simulink model "Gesamt"  (R2015b)
settings: Solver=ode3  SolverMode=SingleTasking  StartTime=0.0  StopTime=inf  RelTol=1e-3
InitFcn:
  | Reglerauslegung
values from neighbouring files (symbols this model uses):
  aMax = 498    [Reglerauslegung.m]
  aMaxPsi = 1    [Reglerauslegung.m]
  Blindzeit = 25    [Reglerauslegung.m]
  dt = 0.005    [Reglerauslegung.m]
  K1 = place(AI1,BI1,pWunschI1)    [Reglerauslegung.m]
  K2 = place(A2,B2,pWunsch2)    [Reglerauslegung.m]
  K3 = place(A3,B3,pWunsch3)    [Reglerauslegung.m]
  Kx = 0.9575    [Reglerauslegung.m]
  Ky = 0.9575    [Reglerauslegung.m]
  Tx = 1/4.1668    (= 0.239992320246)    [Reglerauslegung.m]
  Ty = 1/4.1668    (= 0.239992320246)    [Reglerauslegung.m]
  vMax = 403    [Reglerauslegung.m]
  vMaxPsi = 3    [Reglerauslegung.m]
undefined symbols (not defined in the file or in its folder): sigbuilder_block
libraries: simulink x5, xpcutilitieslib x1
(part 1 of 3)
CloseFcn:
  | rtwprivate ssgencode ModelCloseRequest Robotino_Strecke_reall_2009
settings Model: SimulationMode=external  Creator=atlabor  LastModifiedBy=atlabor
settings SolverCC: EnableConcurrentExecution=on
settings DataIOCC: SignalLoggingSaveFormat=ModelDataLogs
settings OptimizationCC: BlockReduction=off  OptimizeBlockIOStorage=off  BufferReuse=off  GlobalBufferReuse=off  ExpressionFolding=off  ExpressionDepthLimit=2147483647  LocalBlockOutputs=off  InitFltsAndDblsToZero=on
settings DebuggingCC: SaveWithParameterizedLinksMsg=none  UnderspecifiedInitializationDetection=Classic  MergeDetectMultiDrivingBlocksExec=none  SolverPrmCheckMsg=warning  FcnCallInpInsideContextMsg=EnableAllAsWarning  StateNameClashWarn=warning
settings HardwareCC: ProdBitPerPointer=32  ProdLargestAtomicFloat=None  ProdWordSize=32  ProdLongLongMode=on  ProdHWDeviceType=Generic->32-bit x86 compatible
settings SFSimCC: SimParseCustomCode=off
settings RTWCC: SystemTargetFile=TwinCAT.tlc  GenCodeOnly=on  MakeCommand=make_tct  TemplateMakefile=tct_msbuild.tmf  Description=TwinCAT Target  GenerateReport=on  TargetLang=C++
settings STFCustomTargetCC: CompOptLevelCompliant=on  ConcurrentExecutionCompliant=off  GeneratePreprocessorConditionals=Use local settings  MATLABClassNameForMDSCustomization=Simulink.SoftwareTarget.TargetSpecificTriggerConfigurationBase  CPPClassGenCompliant=off  SystemTargetFile=TwinCAT.tlc
settings ConfigComp: CovModelRefEnable=Off  CovSFcnEnable=off

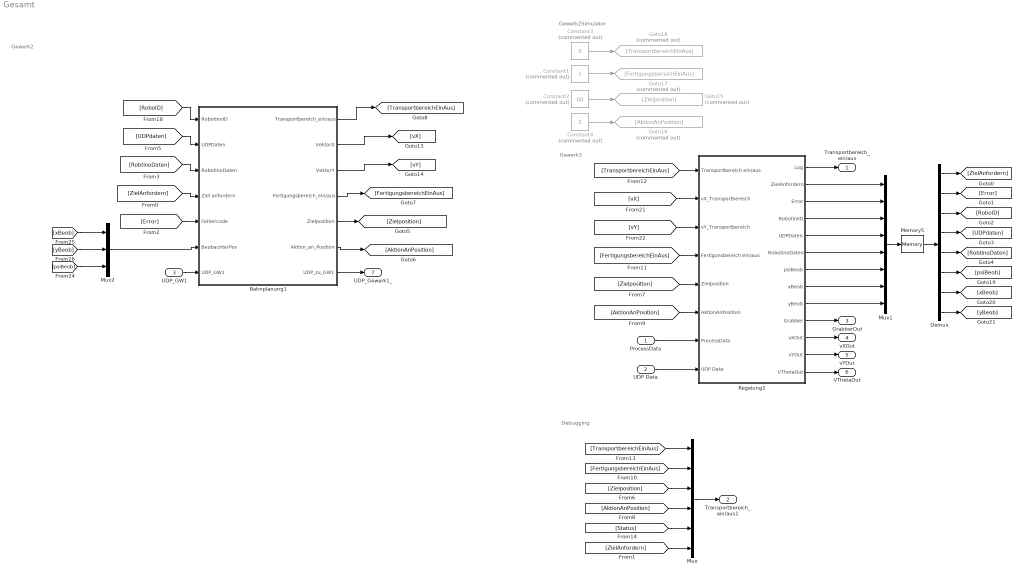
== system Gesamt ==
  note: Gewerk2Simulator
  note: Gewerk3
  note: Gewerk2
  note: Debugging
  ProcessData : Inport
  UDP Data : Inport  Port=2  PortDimensions=56
  UDP_GW1 : Inport  Port=3  PortDimensions=8
  Bahnplanung1 : Subsystem
  Constant1 : Constant  Commented=on
  Constant2 : Constant  Commented=on  Value=60
  Constant3 : Constant  Commented=on  Value=0
  Constant4 : Constant  Commented=on  Value=2
  Demux : Demux  Outputs=8
  Goto15 : Goto  Commented=on  GotoTag=Zielposition
  Goto16 : Goto  Commented=on  GotoTag=AktionAnPosition
  Goto17 : Goto  Commented=on  GotoTag=FertigungsbereichEinAus
  Goto18 : Goto  Commented=on  GotoTag=TransportbereichEinAus
  Memory5 : Memory
  Mux : Mux  Inputs=6
  Mux1 : Mux  Inputs=8
  Mux2 : Mux  Inputs=3
  Regelung1 : Subsystem
  Transportbereich_ein/aus : Outport
  Transportbereich_ein/aus1 : Outport  Port=2
  GrabberOut : Outport  Port=3
  vXOut : Outport  Port=4
  vYOut : Outport  Port=5
  VThetaOut : Outport  Port=6
  UDP_Gewerk1_ : Outport  Port=7
  wires:
  Regelung1/3(Error) -> Mux1/2
  Regelung1/6(RobotinoDaten) -> Mux1/5
  Regelung1/2(ZielAnfordern) -> Mux1/1
  Regelung1/4(RobotiniID) -> Mux1/3
  [ZielAnfordern] -> Mux/6
  Mux1/1 -> Memory5/1
  Demux/1 -> [ZielAnfordern]
  Demux/2 -> [Error]
  Memory5/1 -> Demux/1
  Demux/3 -> [RoboID]
  Demux/4 -> [UDPdaten]
  Regelung1/5(UDPDaten) -> Mux1/4
  Demux/5 -> [RobtinoDaten]
  [Zielposition] -> Mux/3
  [Zielposition] -> Regelung1/5(Zielposition)
  [AktionAnPosition] -> Mux/4
  [AktionAnPosition] -> Regelung1/6(AktionAnPosition)
  [FertigungsbereichEinAus] -> Mux/2
  [FertigungsbereichEinAus] -> Regelung1/4(Fertigunsbereich ein/aus)
  [TransportbereichEinAus] -> Regelung1/1(Transportbereich ein/aus)
  [TransportbereichEinAus] -> Mux/1
  [Status] -> Mux/5
  [RoboID] -> Bahnplanung1/1(RobotinoID)
  [vX] -> Regelung1/2(vX_Transportbereich)
  [vY] -> Regelung1/3(vY_Transportbereich)
  Constant3/1 -> Goto18/1
  Constant1/1 -> Goto17/1
  Constant2/1 -> Goto15/1
  Constant4/1 -> Goto16/1
  Regelung1/7(psiBeob) -> Mux1/6
  Regelung1/8(xBeob) -> Mux1/7
  Regelung1/9(yBeob) -> Mux1/8
  Demux/6 -> [psiBeob]
  Demux/7 -> [xBeob]
  Demux/8 -> [yBeob]
  [psiBeob] -> Mux2/3
  [xBeob] -> Mux2/1
  [yBeob] -> Mux2/2
  Regelung1/1(Log) -> Transportbereich_ein/aus/1
  Mux/1 -> Transportbereich_ein/aus1/1
  [UDPdaten] -> Bahnplanung1/2(UDPDaten)
  [RobtinoDaten] -> Bahnplanung1/3(RobotinoDaten)
  [ZielAnfordern] -> Bahnplanung1/4(Ziel anfordern)
  [Error] -> Bahnplanung1/5(Fehlercode)
  Mux2/1 -> Bahnplanung1/6(BeobachterPos)
  Bahnplanung1/1(Transportbereich_ein/aus) -> [TransportbereichEinAus]
  Bahnplanung1/2(VektorX) -> [vX]
  Bahnplanung1/3("VektorY ") -> [vY]
  Bahnplanung1/4(Fertigungsbereich_ein/aus) -> [FertigungsbereichEinAus]
  Bahnplanung1/5(Zielposition) -> [Zielposition]
  Bahnplanung1/6(Aktion_an_Position) -> [AktionAnPosition]
  ProcessData/1 -> Regelung1/7(ProcessData)
  UDP Data/1 -> Regelung1/8(UDP Data)
  Regelung1/10(Grabber) -> GrabberOut/1
  Regelung1/11(vXOut) -> vXOut/1
  Regelung1/12(vYOut) -> vYOut/1
  Regelung1/13(VThetaOut) -> VThetaOut/1
  Bahnplanung1/7(UDP_zu_GW1) -> UDP_Gewerk1_/1
  UDP_GW1/1 -> Bahnplanung1/7(UDP_GW1)

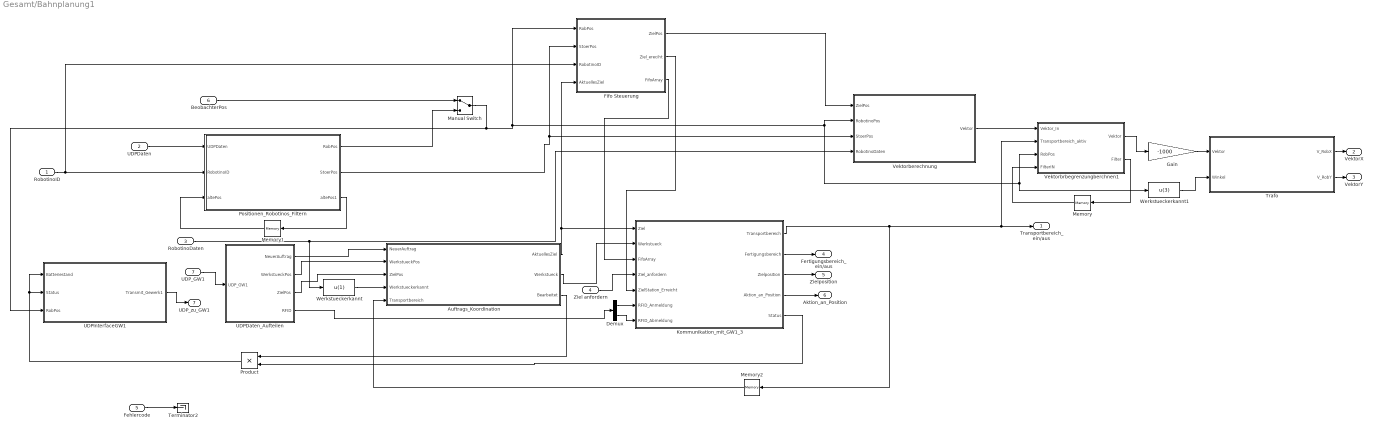
== system Gesamt/Bahnplanung1 ==
  RobotinoID : Inport
  UDPDaten : Inport  Port=2  PortDimensions=56
  RobotinoDaten : Inport  Port=3
  Ziel anfordern : Inport  Port=4
  Fehlercode : Inport  Port=5
  BeobachterPos : Inport  Port=6
  UDP_GW1 : Inport  Port=7  PortDimensions=8
  Auftrags_Koordination : Stateflow chart  TreatAsAtomicUnit=on
  Demux : Demux  Outputs=2
  Fifo Steuerung : Subsystem
  Gain : Gain  Gain=-1000
  Kommunikation_mit_GW1_3 : Stateflow chart  TreatAsAtomicUnit=on
  Manual Switch : ManualSwitch
  Memory : Memory
  Memory1 : Memory
  Memory2 : Memory
  Positionen_Robotinos_Filtern : MATLAB Function  TreatAsAtomicUnit=on
  Product : Product
  Terminator2 : Terminator
  Trafo : MATLAB Function  Tag=Transformation_Global_auf_lokal  TreatAsAtomicUnit=on
  UDPDaten_Aufteilen : Subsystem
  UDPInterfaceGW1 : Subsystem
  Vektorberechnung : Subsystem
  Vektorbrbegrenzungberchnen1 : MATLAB Function  TreatAsAtomicUnit=on
  Werkstueckerkannt : Fcn  Expr=u(1)
  Werkstueckerkannt1 : Fcn  Expr=u(3)
  Transportbereich_ein/aus : Outport
  VektorX : Outport  Port=2  OutDataTypeStr=double
  "VektorY " : Outport  Port=3  OutDataTypeStr=double
  Fertigungsbereich_ein/aus : Outport  Port=4
  Zielposition : Outport  Port=5
  Aktion_an_Position : Outport  Port=6
  UDP_zu_GW1 : Outport  Port=7
  wires:
  RobotinoID/1 -> Positionen_Robotinos_Filtern/2(RobotinoID), Fifo Steuerung/3(RobotinoID)
  UDPDaten/1 -> Positionen_Robotinos_Filtern/1(UDPDaten)
  Positionen_Robotinos_Filtern/2(StoerPos) -> Fifo Steuerung/2(StoerPos), Vektorberechnung/3(StoerPos)
  RobotinoDaten/1 -> Vektorberechnung/4(RobotinoDaten), Werkstueckerkannt/1
  Kommunikation_mit_GW1_3/3(Zielposition) -> Zielposition/1
  Kommunikation_mit_GW1_3/4(Aktion_an_Position) -> Aktion_an_Position/1
  Kommunikation_mit_GW1_3/2(Fertigungsbereich) -> Fertigungsbereich_ein/aus/1
  Kommunikation_mit_GW1_3/1(Transportbereich) -> Memory2/1, Vektorbrbegrenzungberchnen1/2(Transportbereich_aktiv), Transportbereich_ein/aus/1
  UDP_GW1/1 -> UDPDaten_Aufteilen/1(UDP_GW1)
  UDPDaten_Aufteilen/2(WerkstueckPos) -> Auftrags_Koordination/2(WerkstueckPos)
  UDPDaten_Aufteilen/3(ZielPos) -> Auftrags_Koordination/3(ZielPos)
  Auftrags_Koordination/1(AktuellesZiel) -> Fifo Steuerung/4(AktuellesZiel), Kommunikation_mit_GW1_3/1(Ziel)
  Fehlercode/1 -> Terminator2/1
  UDPDaten_Aufteilen/1(NeuerAuftrag) -> Auftrags_Koordination/1(NeuerAuftrag)
  Auftrags_Koordination/2(Werkstueck) -> Kommunikation_mit_GW1_3/2(Werkstueck)
  Werkstueckerkannt/1 -> Auftrags_Koordination/4(Werkstueckerkannt)
  Vektorbrbegrenzungberchnen1/1(Vektor) -> Gain/1
  Gain/1 -> Trafo/1(Vektor)
  Manual Switch/1 -> UDPInterfaceGW1/3(RobPos), Fifo Steuerung/1(RobPos), Vektorbrbegrenzungberchnen1/3(RobPos), Werkstueckerkannt1/1, Vektorberechnung/2(RobotinoPos)
  Vektorberechnung/1(Vektor) -> Vektorbrbegrenzungberchnen1/1(Vektor_In)
  Fifo Steuerung/1(ZielPos) -> Vektorberechnung/1(ZielPos)
  Memory2/1 -> Auftrags_Koordination/5(Transportbereich)
  Kommunikation_mit_GW1_3/5(Status) -> Product/2
  Positionen_Robotinos_Filtern/1(RobPos) -> Manual Switch/2
  Trafo/1(V_RobX) -> VektorX/1
  Trafo/2(V_RobY) -> "VektorY "/1
  BeobachterPos/1 -> Manual Switch/1
  Werkstueckerkannt1/1 -> Trafo/2(Winkel)
  Auftrags_Koordination/3(Bearbeitet) -> Product/1
  Product/1 -> UDPInterfaceGW1/1(Batteriestand), UDPInterfaceGW1/2(Status)
  UDPDaten_Aufteilen/4(RFID) -> Demux/1
  Fifo Steuerung/3("FifoArray ") -> Kommunikation_mit_GW1_3/3(FifoArray)
  Ziel anfordern/1 -> Kommunikation_mit_GW1_3/4(Ziel_anfordern)
  Fifo Steuerung/2(Ziel_ereciht) -> Kommunikation_mit_GW1_3/5(ZielStation_Erreicht)
  Demux/1 -> Kommunikation_mit_GW1_3/6(RFID_Anmeldung)
  Demux/2 -> Kommunikation_mit_GW1_3/7(RFID_Abmeldung)
  Vektorbrbegrenzungberchnen1/2(Filter) -> Memory/1
  Memory/1 -> Vektorbrbegrenzungberchnen1/4(FilterIN)
  Positionen_Robotinos_Filtern/3(altePos1) -> Memory1/1
  Memory1/1 -> Positionen_Robotinos_Filtern/3(altePos)
  UDPInterfaceGW1/1(Transmit_Gewerk1) -> UDP_zu_GW1/1

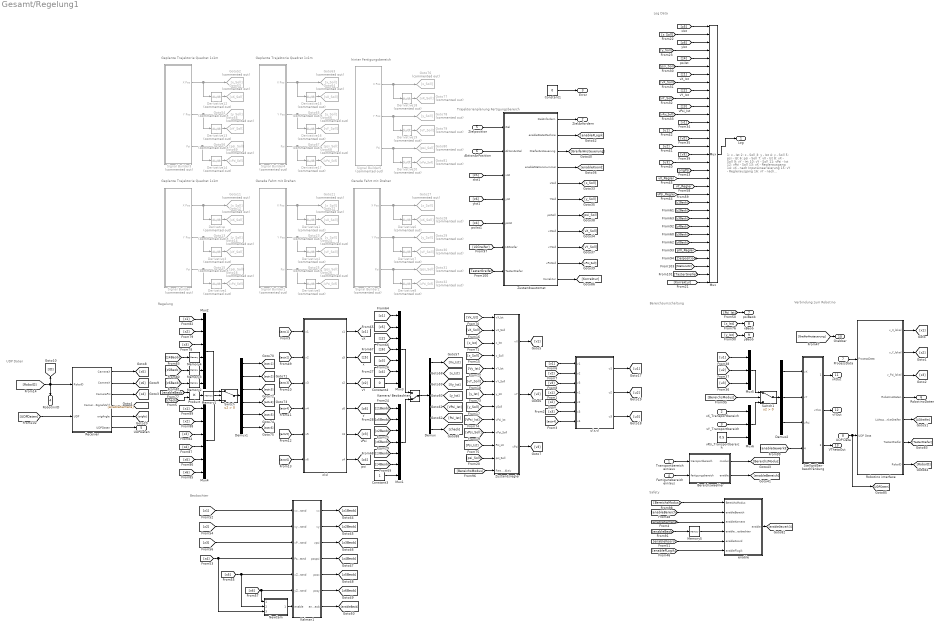
== system Gesamt/Regelung1 ==
  note: Safety
  note: Trajektorienplanung Fertigungsbereich
  note: Regelung
  note: Beobachter
  note: hinter Fertigungsbereich
  note: Geplante Trajektorie Quadrat 1x1m
  note: Geplante Trajektorie Quadrat 1x1m
  note: Gerade Fahrt mit Drehen
  note: Gerade Fahrt mit Drehen
  note: 1:    x     - Ist
      | 2:    x     - Soll
      | 3:    y     - Ist
      | 4:    y     - Soll
      | 5:   psi   - Ist
      | 6:   psi   - Soll
      | 7:   vX   - Ist
      | 8:   vX   - Soll
      | 9:   vY   - Ist
      | 10: vY   - Soll
      | 11: vPsi - Ist
      | 12: vPsi - Soll
      | 13: vX   - Reglerausgang
      | 14: vX   - nach InputLinearisierung
      | 15: vY   - Reglerausgang
      | 16: vY  - nach InputLinearisierung
      | 17: vPsi - Reglerausgang
      | 18: vPsi - nach InputLinearisierung
      | 19: Kamera Psi
      | 20: vX   - Regler (Geschwindigkeit)
      | 21: vY   - Regler (Geschwindigkeit)
      | 22: vPsi - Regler (Geschwindigkeit)
  note: Log Data
  note: Geplante Trajektorie Quadrat 1x1m
  note: UDP Daten
  note: Verbindung zum Robotino
  note: Bereichsumschaltung
  Transportbereich ein/aus : Inport
  vX_Transportbereich : Inport  Port=2
  vY_Transportbereich : Inport  Port=3
  Fertigunsbereich ein/aus : Inport  Port=4
  Zielposition : Inport  Port=5
  AktionAnPosition : Inport  Port=6
  ProcessData : Inport  Port=7
  UDP Data : Inport  Port=8  PortDimensions=56
  Bereichswaehler : MATLAB Function  TreatAsAtomicUnit=on
  Constant1 : Constant  Value=0
  Constant3 : Constant
  Constant4 : Constant  Value=0
  Demux : Demux  Outputs=7
  Demux1 : Demux  Outputs=6
  Demux2 : Demux  Outputs=3
  Derivative{,1..8,12..20} (18 alike) : Derivative  Commented=on
  Goto{11,21,27,52,63,76} (6 alike) : Goto  Commented=on  GotoTag=x_Soll
  Goto{12,22,28,53,64,77} (6 alike) : Goto  Commented=on  GotoTag=vX_Soll
  Goto{13,23,29,54,65,78} (6 alike) : Goto  Commented=on  GotoTag=y_Soll
  Goto{14,24,30,55,66,79} (6 alike) : Goto  Commented=on  GotoTag=vY_Soll
  Goto{15,25,31,56,67,80} (6 alike) : Goto  Commented=on  GotoTag=psi_Soll
  Goto{16,26,32,68..69,81} (6 alike) : Goto  Commented=on  GotoTag=vPsi_Soll
  Kalman1 : MATLAB Function  TreatAsAtomicUnit=on
  Kamera/ Beobachter : ManualSwitch  CurrentSetting=0
  Memory{1..5} (5 alike) : Memory
  Mux : Mux  Inputs=33
  Mux1 : Mux  Inputs=7
  Mux2 : Mux  Inputs=6
  Mux3 : Mux  Inputs=7
  Mux4 : Mux  Inputs=6
  Mux5 : Mux  Inputs=3
  Mux6 : Mux  Inputs=3
  NewCam : MATLAB Function  TreatAsAtomicUnit=on
  Product : Product
  Receiver : Subsystem
  Robotino interface : Subsystem
  Signal Builder : Subsystem  Tag=STV Subsys  Commented=on  LoadFcn=sigbuilder_block('load');  StartFcn=sigbuilder_block('start');  StopFcn=sigbuilder_block('stop');  ClipboardFcn=sigbuilder_block('clipboard');  mask(Sigbuilder block){}
      mask help: Simulink:masks:SigbuilderBlock_MD
      mask init:
      | if ~strcmp(get_param(bdroot(gcbh),'SimulationStatus'),'stopped') tuvar = sigbuilder_block('maskInit'); end
      settings: CopyFcn=sigbuilder_block('copy');  DeleteFcn=sigbuilder_block('delete');  ModelCloseFcn=sigbuilder_block('modelClose');  PreSaveFcn=sigbuilder_block('preSave');  PauseFcn=sigbuilder_block('pause');  ContinueFcn=sigbuilder_block('continue');  NameChangeFcn=sigbuilder_block('namechange');  OpenFcn=sigbuilder_block('open',[6 30 1248 660 ]);  CloseFcn=sigbuilder_block('close');
      mask Display: plot(0, 0, 100, 100,[2, 2, 32, 32, 2], [68, 8, 8, 68, 68],[32, 2], [38, 38], [32, 19, 2],[53, 60, 44], [32, 17, 17, 2],[16, 16, 31, 31]);txt = getActiveGroup(gcbh);text(2, 100, txt,'verticalAlignment', 'top');
  Signal Builder1 : Subsystem  Tag=STV Subsys  Commented=on  LoadFcn=sigbuilder_block('load');  StartFcn=sigbuilder_block('start');  StopFcn=sigbuilder_block('stop');  ClipboardFcn=sigbuilder_block('clipboard');  mask(Sigbuilder block){}
      mask help: Simulink:masks:SigbuilderBlock_MD
      mask init:
      | if ~strcmp(get_param(bdroot(gcbh),'SimulationStatus'),'stopped') tuvar = sigbuilder_block('maskInit'); end
      settings: CopyFcn=sigbuilder_block('copy');  DeleteFcn=sigbuilder_block('delete');  ModelCloseFcn=sigbuilder_block('modelClose');  PreSaveFcn=sigbuilder_block('preSave');  PauseFcn=sigbuilder_block('pause');  ContinueFcn=sigbuilder_block('continue');  NameChangeFcn=sigbuilder_block('namechange');  OpenFcn=sigbuilder_block('open',[6.06316 30.3158 1248.25 659.368 ]);  CloseFcn=sigbuilder_block('close');
      mask Display: plot(0, 0, 100, 100,[2, 2, 32, 32, 2], [68, 8, 8, 68, 68],[32, 2], [38, 38], [32, 19, 2],[53, 60, 44], [32, 17, 17, 2],[16, 16, 31, 31]);txt = getActiveGroup(gcbh);text(2, 100, txt,'verticalAlignment', 'top');
  Signal Builder2 : Subsystem  Tag=STV Subsys  Commented=on  LoadFcn=sigbuilder_block('load');  StartFcn=sigbuilder_block('start');  StopFcn=sigbuilder_block('stop');  ClipboardFcn=sigbuilder_block('clipboard');  mask(Sigbuilder block){}
      mask help: Simulink:masks:SigbuilderBlock_MD
      mask init:
      | if ~strcmp(get_param(bdroot(gcbh),'SimulationStatus'),'stopped') tuvar = sigbuilder_block('maskInit'); end
      settings: CopyFcn=sigbuilder_block('copy');  DeleteFcn=sigbuilder_block('delete');  ModelCloseFcn=sigbuilder_block('modelClose');  PreSaveFcn=sigbuilder_block('preSave');  PauseFcn=sigbuilder_block('pause');  ContinueFcn=sigbuilder_block('continue');  NameChangeFcn=sigbuilder_block('namechange');  OpenFcn=sigbuilder_block('open',[6 30 1248 660 ]);  CloseFcn=sigbuilder_block('close');
      mask Display: plot(0, 0, 100, 100,[2, 2, 32, 32, 2], [68, 8, 8, 68, 68],[32, 2], [38, 38], [32, 19, 2],[53, 60, 44], [32, 17, 17, 2],[16, 16, 31, 31]);txt = getActiveGroup(gcbh);text(2, 100, txt,'verticalAlignment', 'top');
  Signal Builder3 : Subsystem  Tag=STV Subsys  Commented=on  LoadFcn=sigbuilder_block('load');  StartFcn=sigbuilder_block('start');  StopFcn=sigbuilder_block('stop');  ClipboardFcn=sigbuilder_block('clipboard');  mask(Sigbuilder block){}
      mask help: Simulink:masks:SigbuilderBlock_MD
      mask init:
      | if ~strcmp(get_param(bdroot(gcbh),'SimulationStatus'),'stopped') tuvar = sigbuilder_block('maskInit'); end
      settings: CopyFcn=sigbuilder_block('copy');  DeleteFcn=sigbuilder_block('delete');  ModelCloseFcn=sigbuilder_block('modelClose');  PreSaveFcn=sigbuilder_block('preSave');  PauseFcn=sigbuilder_block('pause');  ContinueFcn=sigbuilder_block('continue');  NameChangeFcn=sigbuilder_block('namechange');  OpenFcn=sigbuilder_block('open',[6 30 1248 660 ]);  CloseFcn=sigbuilder_block('close');
      mask Display: plot(0, 0, 100, 100,[2, 2, 32, 32, 2], [68, 8, 8, 68, 68],[32, 2], [38, 38], [32, 19, 2],[53, 60, 44], [32, 17, 17, 2],[16, 16, 31, 31]);txt = getActiveGroup(gcbh);text(2, 100, txt,'verticalAlignment', 'top');
  Signal Builder4 : Subsystem  Tag=STV Subsys  Commented=on  LoadFcn=sigbuilder_block('load');  StartFcn=sigbuilder_block('start');  StopFcn=sigbuilder_block('stop');  ClipboardFcn=sigbuilder_block('clipboard');  mask(Sigbuilder block){}
      mask help: Simulink:masks:SigbuilderBlock_MD
      mask init:
      | if ~strcmp(get_param(bdroot(gcbh),'SimulationStatus'),'stopped') tuvar = sigbuilder_block('maskInit'); end
      settings: CopyFcn=sigbuilder_block('copy');  DeleteFcn=sigbuilder_block('delete');  ModelCloseFcn=sigbuilder_block('modelClose');  PreSaveFcn=sigbuilder_block('preSave');  PauseFcn=sigbuilder_block('pause');  ContinueFcn=sigbuilder_block('continue');  NameChangeFcn=sigbuilder_block('namechange');  OpenFcn=sigbuilder_block('open',[6 30 1248 660 ]);  CloseFcn=sigbuilder_block('close');
      mask Display: plot(0, 0, 100, 100,[2, 2, 32, 32, 2], [68, 8, 8, 68, 68],[32, 2], [38, 38], [32, 19, 2],[53, 60, 44], [32, 17, 17, 2],[16, 16, 31, 31]);txt = getActiveGroup(gcbh);text(2, 100, txt,'verticalAlignment', 'top');
  Signal Builder5 : Subsystem  Tag=STV Subsys  Commented=on  LoadFcn=sigbuilder_block('load');  StartFcn=sigbuilder_block('start');  StopFcn=sigbuilder_block('stop');  ClipboardFcn=sigbuilder_block('clipboard');  mask(Sigbuilder block){}
      mask help: Simulink:masks:SigbuilderBlock_MD
      mask init:
      | if ~strcmp(get_param(bdroot(gcbh),'SimulationStatus'),'stopped') tuvar = sigbuilder_block('maskInit'); end
      settings: CopyFcn=sigbuilder_block('copy');  DeleteFcn=sigbuilder_block('delete');  ModelCloseFcn=sigbuilder_block('modelClose');  PreSaveFcn=sigbuilder_block('preSave');  PauseFcn=sigbuilder_block('pause');  ContinueFcn=sigbuilder_block('continue');  NameChangeFcn=sigbuilder_block('namechange');  OpenFcn=sigbuilder_block('open',[6 30 1248 660 ]);  CloseFcn=sigbuilder_block('close');
      mask Display: plot(0, 0, 100, 100,[2, 2, 32, 32, 2], [68, 8, 8, 68, 68],[32, 2], [38, 38], [32, 19, 2],[53, 60, 44], [32, 17, 17, 2],[16, 16, 31, 31]);txt = getActiveGroup(gcbh);text(2, 100, txt,'verticalAlignment', 'top');
  "Stellgrößen- beschränkung " : Subsystem
  Switch : Switch  Criteria=u2 > Threshold
  Switch1 : Switch  Criteria=u2 > Threshold
  Zustandsautomat : Subsystem
  Zustandsregler : Subsystem
  "enable " : MATLAB Function  TreatAsAtomicUnit=on
  "u(x,v) " : MATLAB Function  TreatAsAtomicUnit=on
  vPsi_Transportbereich : Constant  Value=0.5
  z(x) : MATLAB Function  TreatAsAtomicUnit=on
  Log : Outport
  ZielAnfordern : Outport  Port=2
  Error : Outport  Port=3
  RobotiniID : Outport  Port=4
  UDPDaten : Outport  Port=5
  RobotinoDaten : Outport  Port=6
  psiBeob : Outport  Port=7
  xBeob : Outport  Port=8
  yBeob : Outport  Port=9
  Grabber : Outport  Port=10
  vXOut : Outport  Port=11
  vYOut : Outport  Port=12
  VThetaOut : Outport  Port=13
  wires:
  [TasterGreifer] -> Zustandsautomat/7("TasterGreifer ")
  Robotino interface/6(TasterGreifer) -> [TasterGreifer]
  [y_Ist] -> yBeob/1
  [x_Ist] -> xBeob/1
  [Psi_Ist] -> psiBeob/1
  Zustandsautomat/1(ZielAnfordern) -> ZielAnfordern/1
  [z4] -> Zustandsautomat/5(psiIst)
  [z5] -> Zustandsautomat/3(xIst)
  Zustandsautomat/6(YSoll) -> [y_Soll]
  Zustandsautomat/9(vYSoll) -> [vY_Soll]
  Zustandsautomat/5(xSoll) -> [x_Soll]
  Zustandsautomat/8(vXSoll) -> [vX_Soll]
  Zustandsautomat/10(vPsiSoll) -> [vPsi_Soll]
  Zustandsautomat/4(enableStationsnummer) -> [enableKoord]
  [z6] -> Zustandsautomat/4(yIst)
  Zustandsautomat/2(enableStateMachine) -> [enableFLogik]
  Zustandsautomat/7(psiSoll) -> [psi_Soll]
  Zustandsautomat/3(GreiferAnsteuerung) -> [GreiferAnsteuerung]
  [x_Soll] -> Zustandsregler/4(x_Soll)
  Switch/1 -> Demux1/1
  Mux3/1 -> Kamera/ Beobachter/1
  z(x)/5(z3) -> [z3]
  Kalman1/7(enableBeob) -> [enableBeob]
  [actx6] -> z(x)/6(x6)
  [x6] -> Kalman1/6(yZustand), NewCam/1(yZustand)
  [y_Soll] -> Zustandsregler/8(ySoll)
  Mux2/1 -> Switch/1
  Memory4/1 -> Mux2/4
  Demux1/3 -> [actx3]
  Memory1/1 -> Switch/2
  z(x)/4(z6) -> [z6]
  Demux1/2 -> [actx2]
  z(x)/2(z5) -> [z5]
  Demux/5 -> [VPsi_Ist]
  [x5] -> Mux4/5
  [x1] -> Mux2/1
  Kamera/ Beobachter/1 -> Demux/1
  Constant3/1 -> Mux1/7
  [z4Beob] -> Memory4/1
  Kalman1/4(pospsi) -> [z4Beob]
  [actx5] -> z(x)/5(x5)
  Demux/4 -> [y_Ist]
  z(x)/3(z2) -> [z2]
  Demux1/4 -> [actx4]
  Demux1/5 -> [actx5]
  [vY_Soll] -> Zustandsregler/6("vY_Soll ")
  Product/1 -> Memory1/1
  [z6Beob] -> Memory2/1
  [psi_Soll] -> Zustandsregler/12("psi_Soll ")
  Demux/2 -> [x_Ist]
  [Vx_Ist] -> Zustandsregler/1(vX_Ist)
  [vPsi_Soll] -> Zustandsregler/10(vPsi_Soll)
  Zustandsregler/1(vX) -> [v1]
  [z3] -> Mux3/5
  Demux1/6 -> [actx6]
  [x_Ist] -> Zustandsregler/3(x_Ist)
  [actx4] -> z(x)/4(x4)
  [actx2] -> z(x)/2(x2)
  [x3] -> Mux2/3
  "u(x,v) "/1(u1) -> [u1]
  Demux/7 -> [check]
  z(x)/6(z4) -> [z4]
  [z4Beob] -> Mux1/6
  Kalman1/1(vx) -> [z1Beob]
  [x6] -> Mux4/6
  z(x)/1(z1) -> [z1]
  Zustandsregler/3("vPsi ") -> [v3]
  [Vy_Ist] -> Zustandsregler/5(vY_Ist)
  [v3] -> "u(x,v) "/3(v3)
  [v2] -> "u(x,v) "/2(v2)
  [x2] -> Mux2/2
  [y_Ist] -> Zustandsregler/7(y_Ist)
  [z5Beob] -> Mux1/2
  [x2] -> "u(x,v) "/5(x2)
  [actx1] -> z(x)/1(x1)
  [Psi_Ist] -> Zustandsregler/11(Psi_ist)
  Mux4/1 -> Switch/3
  "u(x,v) "/2(u2) -> [u2]
  Demux/6 -> [Psi_Ist]
  [VPsi_Ist] -> Zustandsregler/9(vPsi_ist)
  [x3] -> "u(x,v) "/6(x3)
  Kalman1/3(vpsi) -> [z3Beob]
  [z6Beob] -> Mux1/4
  [x3] -> Mux4/3
  Mux1/1 -> Kamera/ Beobachter/2
  [z1] -> Mux3/1
  [z6] -> Mux3/4
  [actx4] -> "u(x,v) "/7(x4)
  [z4] -> Mux3/6
  [v1] -> "u(x,v) "/1(v1)
  Kalman1/6(posy) -> [z6Beob]
  [z2] -> Mux3/3
  [enableBeob] -> Product/1
  Memory2/1 -> Mux2/6
  [x1] -> Mux4/1
  Demux/3 -> [Vy_Ist]
  NewCam/1(enable) -> Kalman1/7(enable)
  [check] -> Product/2
  [z1] -> Kalman1/1(vxZustand)
  [x2] -> Mux4/2
  [vX_Soll] -> Zustandsregler/2("vX_Soll ")
  [z3Beob] -> Mux1/5
  Memory3/1 -> Mux2/5
  Kalman1/5(posx) -> [z5Beob]
  [z5] -> Mux3/2
  "u(x,v) "/3(u3) -> [u3]
  [actx3] -> z(x)/3(x3)
  [x1] -> "u(x,v) "/4(x1)
  [z2Beob] -> Mux1/3
  [z5Beob] -> Memory3/1
  [z1Beob] -> Mux1/1
  [x4] -> Kalman1/4(PsiZustand), NewCam/3(psiZustand)
  Zustandsregler/2(vY) -> [v2]
  [x5] -> Kalman1/5(xZustand), NewCam/2(xZustand)
  [z2] -> Kalman1/2(vyZustand)
  Demux/1 -> [Vx_Ist]
  Demux1/1 -> [actx1]
  [x4] -> Mux4/4
  Constant4/1 -> Mux3/7
  [z3] -> Kalman1/3(vPsiZustand)
  Kalman1/2(vy) -> [z2Beob]
  Switch1/1 -> Demux2/1
  Robotino interface/4("RobotinoDaten ") -> RobotinoDaten/1
  Receiver/6(UDPDaten) -> UDPDaten/1
  Derivative1/1 -> Goto22/1
  Signal Builder1/3(Psi) -> Goto25/1, Derivative5/1
  Signal Builder2/1(X Pos) -> Goto27/1, Derivative6/1
  Demux2/1 -> "Stellgrößen- beschränkung "/1(vX)
  Derivative5/1 -> Goto26/1
  Signal Builder5/2(Y Pos) -> Derivative19/1, Goto78/1
  Signal Builder2/2(Y Pos) -> Goto29/1, Derivative7/1
  Derivative6/1 -> Goto28/1
  Derivative3/1 -> Goto14/1
  Signal Builder/3(Psi) -> Goto15/1, Derivative4/1
  Derivative2/1 -> Goto24/1
  Derivative13/1 -> Goto55/1
  Derivative16/1 -> Goto66/1
  Derivative17/1 -> Goto68/1
  Derivative15/1 -> Goto64/1
  Signal Builder5/1(X Pos) -> Derivative18/1, Goto76/1
  Signal Builder/2(Y Pos) -> Goto13/1, Derivative3/1
  Derivative8/1 -> Goto32/1
  Derivative14/1 -> Goto69/1
  Derivative12/1 -> Goto53/1
  Derivative20/1 -> Goto81/1
  Derivative19/1 -> Goto79/1
  Derivative18/1 -> Goto77/1
  Robotino interface/1(v_X_lokal) -> [x1]
  Signal Builder3/1(X Pos) -> Derivative12/1, Goto52/1
  Receiver/2(CameraY) -> [x6]
  Receiver/1(CameraX) -> [x5]
  Signal Builder4/2(Y Pos) -> Derivative16/1, Goto65/1
  Zielposition/1 -> Zustandsautomat/1("Ziel ")
  Signal Builder4/1(X Pos) -> Derivative15/1, Goto63/1
  AktionAnPosition/1 -> Zustandsautomat/2(AktionAnZiel)
  Derivative/1 -> Goto12/1
  Signal Builder3/2(Y Pos) -> Derivative13/1, Goto54/1
  vY_Transportbereich/1 -> Mux6/2
  Robotino interface/2("v_Y_lokal ") -> [x2]
  Robotino interface/3("v_Psi_lokal ") -> [x3]
  Signal Builder4/3(Psi) -> Derivative17/1, Goto67/1
  vX_Transportbereich/1 -> Mux6/1
  Receiver/3("CameraPsi ") -> [x4]
  Receiver/4(CameraSignalValid) -> [enableKamera]
  Signal Builder1/2(Y Pos) -> Goto23/1, Derivative2/1
  Signal Builder3/3(Psi) -> Derivative14/1, Goto56/1
  Derivative7/1 -> Goto30/1
  Signal Builder2/3(Psi) -> Goto31/1, Derivative8/1
  Signal Builder1/1(X Pos) -> Goto21/1, Derivative1/1
  Signal Builder5/3(Psi) -> Derivative20/1, Goto80/1
  Demux2/3 -> "Stellgrößen- beschränkung "/3(vPsi)
  Demux2/2 -> "Stellgrößen- beschränkung "/2(vY)
  Receiver/5("origAngle ") -> [origPsi]
  Mux6/1 -> Switch1/3
  Transportbereich ein/aus/1 -> Bereichswaehler/1(transportbereich)
  vPsi_Transportbereich/1 -> Mux6/3
  [u3] -> Mux5/3
  [u2] -> Mux5/2
  Signal Builder/1(X Pos) -> Goto11/1, Derivative/1
  Derivative4/1 -> Goto16/1
  [u1] -> Mux5/1
  Mux5/1 -> Switch1/1
  Constant1/1 -> Error/1
  Bereichswaehler/2(enable) -> [enableBereich]
  Fertigunsbereich ein/aus/1 -> Bereichswaehler/2(fertigungsbereich)
  Bereichswaehler/1(modus) -> [BereichsModus]
  [BereichsModus] -> Switch1/2
  [BereichsModus] -> Zustandsregler/13(Fertigungsbereich Aktiv)
  Robotino interface/5(LichtschrankeGreifer) -> [LSGreifer]
  [LSGreifer] -> Zustandsautomat/6("LSGreifer ")
  [enableBeob] -> Memory5/1
  Memory5/1 -> "enable "/4(enableBeobachter)
  [enableKamera] -> "enable "/3(enableKamera)
  [enableBereich] -> "enable "/2(enableBereich)
  [BereichsModus] -> "enable "/1(BereichsModus)
  [enableKoord] -> "enable "/5(enableKoord)
  [enableFLogik] -> "enable "/6(enableFlogik)
  "enable "/1(enable) -> [enableGewerk3]
  [GreiferAnsteuerung] -> Grabber/1
  "Stellgrößen- beschränkung "/1(vXlim) -> vXOut/1
  "Stellgrößen- beschränkung "/2(vYlim) -> vYOut/1
  "Stellgrößen- beschränkung "/3(vPsiLim) -> VThetaOut/1
  ProcessData/1 -> Robotino interface/1(ProcessData)
  UDP Data/1 -> [UDPDaten], Robotino interface/2(UDP Data)
  [enableGewerk3] -> "Stellgrößen- beschränkung "/4(enableGewerk3)
  Robotino interface/7(RoboID) -> [RoboID]
  [RoboID] -> [ID], RobotiniID/1, Receiver/1("RoboID ")
  [UDPDaten] -> Receiver/2(UDP)
  Zustandsautomat/11(Korrektur) -> [Korrektur]
  [TasterGreifer] -> Mux/32
  [pXI_Regler] -> Mux/29
  [vX_Regler] -> Mux/20
  [z4] -> Mux/5
  [y_Soll] -> Mux/4
  [z1Beob] -> Mux/23
  [v2] -> Mux/15
  [v1] -> Mux/13
  [psi_Soll] -> Mux/6
  [vPsi_Regler] -> Mux/22
  [x_Soll] -> Mux/2
  [z5Beob] -> Mux/27
  [z4Beob] -> Mux/26
  [vY_Regler] -> Mux/21
  [z3Beob] -> Mux/25
  [z2] -> Mux/9
  [z3] -> Mux/11
  [vX_Soll] -> Mux/8
  [vY_Soll] -> Mux/10
  [z6Beob] -> Mux/28
  [z2Beob] -> Mux/24
  [vPsi_Soll] -> Mux/12
  [z6] -> Mux/3
  [v3] -> Mux/17
  [z5] -> Mux/1
  [origPsi] -> Mux/19
  [u1] -> Mux/14
  [u3] -> Mux/18
  [u2] -> Mux/16
  [z1] -> Mux/7
  Mux/1 -> Log/1
  [Zielposition] -> Mux/30
  [StationsNr] -> Mux/31
  [Korrektur] -> Mux/33

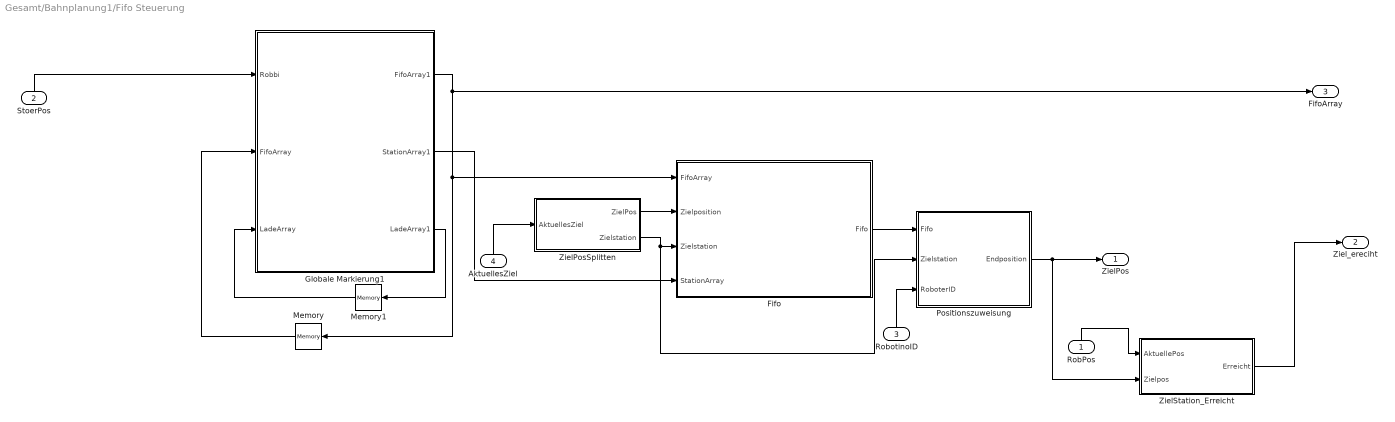
== system Gesamt/Bahnplanung1/Fifo Steuerung ==
  RobPos : Inport  PortDimensions=3
  StoerPos : Inport  Port=2  PortDimensions=15
  RobotinoID : Inport  Port=3
  AktuellesZiel : Inport  Port=4
  Fifo : Stateflow chart  TreatAsAtomicUnit=on
  Globale Markierung1 : MATLAB Function  TreatAsAtomicUnit=on
  Memory : Memory
  Memory1 : Memory
  Positionszuweisung : MATLAB Function  TreatAsAtomicUnit=on
  ZielPosSplitten : MATLAB Function  TreatAsAtomicUnit=on
  ZielStation_Erreicht : MATLAB Function  TreatAsAtomicUnit=on
  ZielPos : Outport  PortDimensions=[1 2]
  Ziel_ereciht : Outport  Port=2
  "FifoArray " : Outport  Port=3
  wires:
  RobotinoID/1 -> Positionszuweisung/3(RoboterID)
  RobPos/1 -> ZielStation_Erreicht/1(AktuellePos)
  StoerPos/1 -> Globale Markierung1/1(Robbi)
  AktuellesZiel/1 -> ZielPosSplitten/1(AktuellesZiel)
  Positionszuweisung/1(Endposition) -> ZielStation_Erreicht/2(Zielpos), ZielPos/1
  Globale Markierung1/2(StationArray1) -> Fifo/4(StationArray)
  ZielPosSplitten/1(ZielPos) -> Fifo/2(Zielposition)
  ZielPosSplitten/2(Zielstation) -> Positionszuweisung/2(Zielstation), Fifo/3(Zielstation)
  Memory/1 -> Globale Markierung1/2(FifoArray)
  Globale Markierung1/3(LadeArray1) -> Memory1/1
  Memory1/1 -> Globale Markierung1/3(LadeArray)
  ZielStation_Erreicht/1(Erreicht) -> Ziel_ereciht/1
  Fifo/1(Fifo) -> Positionszuweisung/1(Fifo)
  Globale Markierung1/1(FifoArray1) -> Memory/1, Fifo/1(FifoArray), "FifoArray "/1

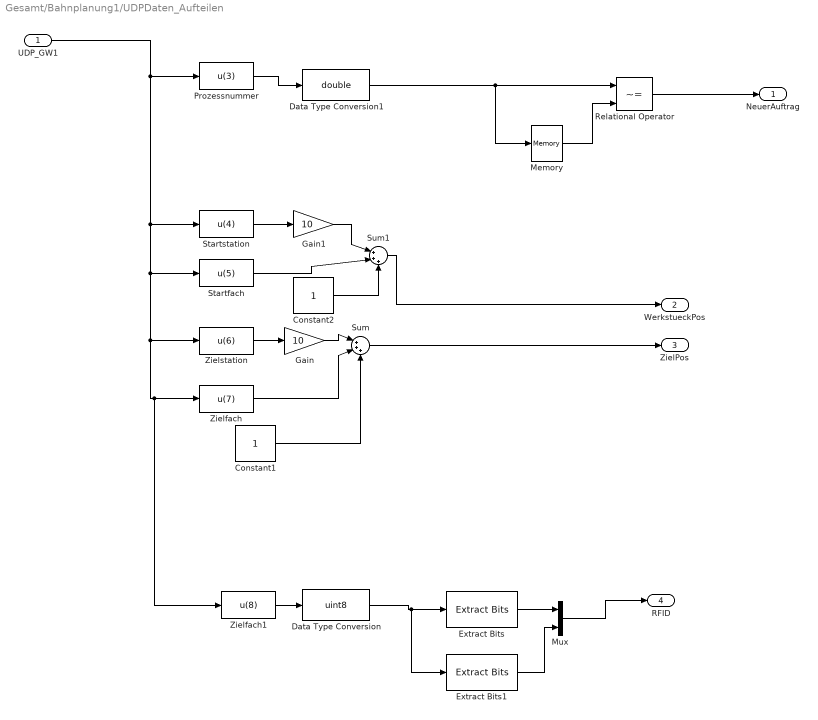
== system Gesamt/Bahnplanung1/UDPDaten_Aufteilen ==
  UDP_GW1 : Inport  PortDimensions=8
  Constant1 : Constant
  Constant2 : Constant
  Data Type Conversion : DataTypeConversion  OutDataTypeStr=uint8
  Data Type Conversion1 : DataTypeConversion  OutDataTypeStr=double
  Extract Bits : simulink/Logic and Bit Operations/Extract Bits  bitsToExtract=Range of bits  numBits=8  bitIdxRange=[0]  outScalingMode=Treat bit field as an integer
  Extract Bits1 : simulink/Logic and Bit Operations/Extract Bits  bitsToExtract=Range of bits  numBits=8  bitIdxRange=[1]  outScalingMode=Treat bit field as an integer
  Gain : Gain  Gain=10
  Gain1 : Gain  Gain=10
  Memory : Memory
  Mux : Mux  Inputs=2
  Prozessnummer : Fcn  Expr=u(3)
  Relational Operator : RelationalOperator  Operator=~=  OutDataTypeStr=boolean
  Startfach : Fcn  Expr=u(5)
  Startstation : Fcn  Expr=u(4)
  Sum : Sum  Inputs=|+++
  Sum1 : Sum  Inputs=|+++
  Zielfach : Fcn  Expr=u(7)
  Zielfach1 : Fcn  Expr=u(8)
  Zielstation : Fcn  Expr=u(6)
  NeuerAuftrag : Outport
  WerkstueckPos : Outport  Port=2
  ZielPos : Outport  Port=3
  RFID : Outport  Port=4
  wires:
  Zielfach/1 -> Sum/2
  Gain/1 -> Sum/1
  Zielstation/1 -> Gain/1
  UDP_GW1/1 -> Prozessnummer/1, Zielfach1/1, Zielfach/1, Zielstation/1, Startfach/1, Startstation/1
  Sum1/1 -> WerkstueckPos/1
  Startfach/1 -> Sum1/2
  Gain1/1 -> Sum1/1
  Constant2/1 -> Sum1/3
  Startstation/1 -> Gain1/1
  Constant1/1 -> Sum/3
  Sum/1 -> ZielPos/1
  Relational Operator/1 -> NeuerAuftrag/1
  Zielfach1/1 -> Data Type Conversion/1
  Data Type Conversion/1 -> Extract Bits1/1, Extract Bits/1
  Data Type Conversion1/1 -> Memory/1, Relational Operator/1
  Memory/1 -> Relational Operator/2
  Extract Bits1/1 -> Mux/2
  Mux/1 -> RFID/1
  Prozessnummer/1 -> Data Type Conversion1/1
  Extract Bits/1 -> Mux/1

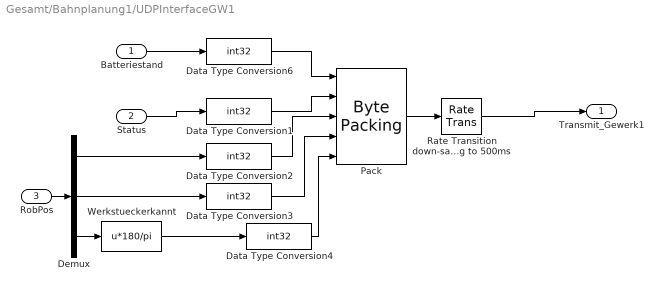
== system Gesamt/Bahnplanung1/UDPInterfaceGW1 ==
  Batteriestand : Inport
  Status : Inport  Port=2
  RobPos : Inport  Port=3
  Data Type Conversion{1..4,6} (5 alike) : DataTypeConversion  OutDataTypeStr=int32
  Demux : Demux  Outputs=3
  Pack : xpcutilitieslib/Byte Packing   MaskPackedDataType=uint8  MaskUnpackedDataTypes={'int32','int32','int32','int32','int32'}  MaskAlignment=1
  Rate Transition down-sampling to 500ms : RateTransition  OutPortSampleTime=0.5
  Werkstueckerkannt : Fcn  Expr=u*180/pi
  Transmit_Gewerk1 : Outport
  wires:
  Pack/1 -> Rate Transition down-sampling to 500ms/1
  Data Type Conversion1/1 -> Pack/2
  Data Type Conversion6/1 -> Pack/1
  Batteriestand/1 -> Data Type Conversion6/1
  Status/1 -> Data Type Conversion1/1
  Rate Transition down-sampling to 500ms/1 -> Transmit_Gewerk1/1
  Data Type Conversion2/1 -> Pack/3
  Data Type Conversion3/1 -> Pack/4
  Data Type Conversion4/1 -> Pack/5
  RobPos/1 -> Demux/1
  Demux/1 -> Data Type Conversion2/1
  Demux/2 -> Data Type Conversion3/1
  Demux/3 -> Werkstueckerkannt/1
  Werkstueckerkannt/1 -> Data Type Conversion4/1

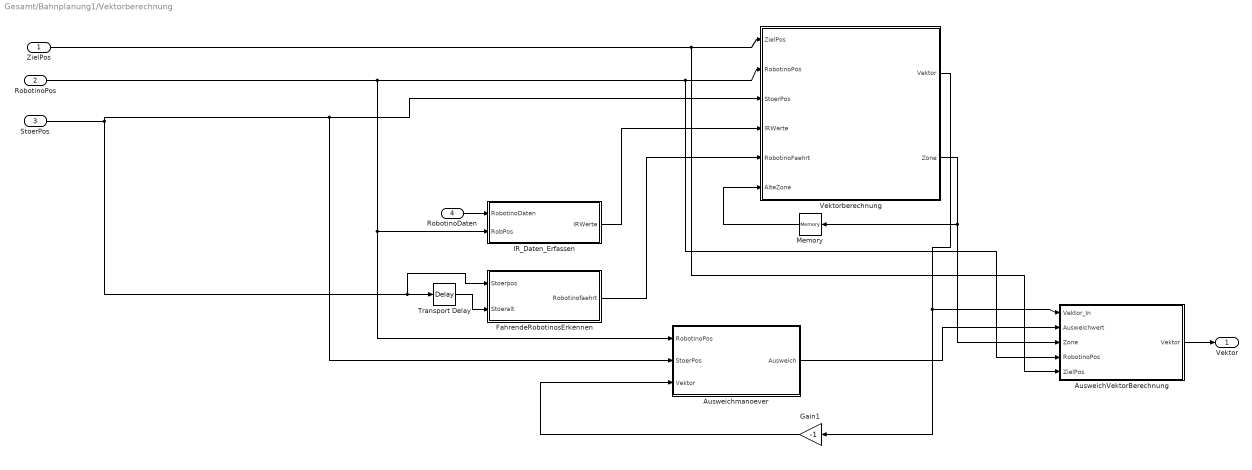
== system Gesamt/Bahnplanung1/Vektorberechnung ==
  ZielPos : Inport
  RobotinoPos : Inport  Port=2
  StoerPos : Inport  Port=3
  RobotinoDaten : Inport  Port=4  PortDimensions=15
  AusweichVektorBerechnung : MATLAB Function  TreatAsAtomicUnit=on
  Ausweichmanoever : MATLAB Function  TreatAsAtomicUnit=on
  FahrendeRobotinosErkennen : MATLAB Function  TreatAsAtomicUnit=on
  Gain1 : Gain  Gain=-1
  IR_Daten_Erfassen : MATLAB Function  TreatAsAtomicUnit=on
  Memory : Memory
  Transport Delay : TransportDelay
  Vektorberechnung : MATLAB Function  TreatAsAtomicUnit=on
  Vektor : Outport
  wires:
  RobotinoPos/1 -> AusweichVektorBerechnung/4(RobotinoPos), Vektorberechnung/2(RobotinoPos), IR_Daten_Erfassen/2(RobPos), Ausweichmanoever/1(RobotinoPos)
  RobotinoDaten/1 -> IR_Daten_Erfassen/1(RobotinoDaten)
  StoerPos/1 -> Transport Delay/1, FahrendeRobotinosErkennen/1(Stoerpos), Vektorberechnung/3(StoerPos), Ausweichmanoever/2(StoerPos)
  ZielPos/1 -> AusweichVektorBerechnung/5(ZielPos), Vektorberechnung/1(ZielPos)
  Ausweichmanoever/1(Ausweich) -> AusweichVektorBerechnung/2(Ausweichwert)
  Vektorberechnung/1(Vektor) -> Gain1/1, AusweichVektorBerechnung/1(Vektor_In)
  Gain1/1 -> Ausweichmanoever/3(Vektor)
  IR_Daten_Erfassen/1(IRWerte) -> Vektorberechnung/4(IRWerte)
  AusweichVektorBerechnung/1(Vektor) -> Vektor/1
  Vektorberechnung/2(Zone) -> AusweichVektorBerechnung/3(Zone), Memory/1
  FahrendeRobotinosErkennen/1(Robotinofaehrt) -> Vektorberechnung/5(RobotinoFaehrt)
  Transport Delay/1 -> FahrendeRobotinosErkennen/2(Stoeralt)
  Memory/1 -> Vektorberechnung/6(AlteZone)

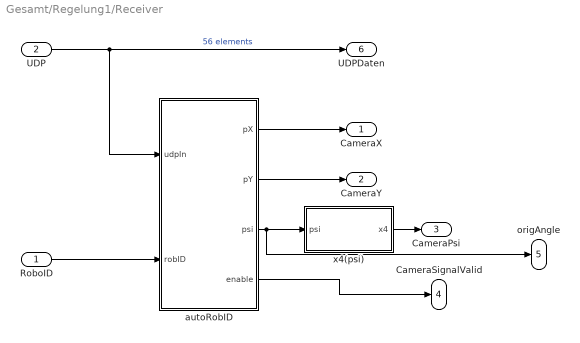
== system Gesamt/Regelung1/Receiver ==
  "RoboID " : Inport
  UDP : Inport  Port=2
  autoRobID : MATLAB Function  TreatAsAtomicUnit=on
  x4(psi) : MATLAB Function  TreatAsAtomicUnit=on
  CameraX : Outport
  CameraY : Outport  Port=2
  "CameraPsi " : Outport  Port=3
  CameraSignalValid : Outport  Port=4
  "origAngle " : Outport  Port=5
  UDPDaten : Outport  Port=6
  wires:
  "RoboID "/1 -> autoRobID/2(robID)
  UDP/1 -> autoRobID/1(udpIn), UDPDaten/1  "56 elements"
  autoRobID/3(psi) -> x4(psi)/1(psi), "origAngle "/1
  autoRobID/2(pY) -> CameraY/1
  x4(psi)/1(x4) -> "CameraPsi "/1
  autoRobID/1(pX) -> CameraX/1
  autoRobID/4(enable) -> CameraSignalValid/1

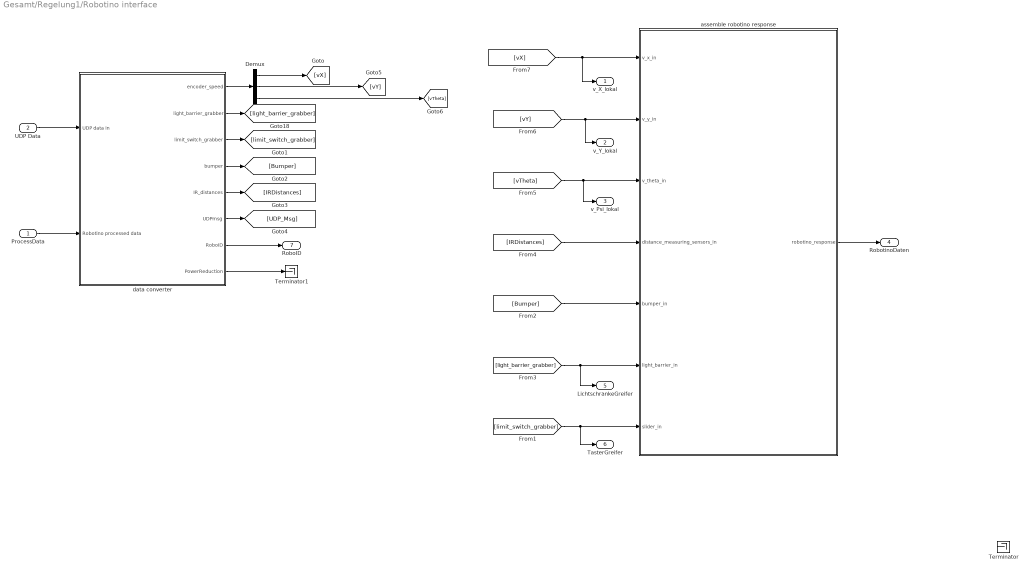
== system Gesamt/Regelung1/Robotino interface ==
  ProcessData : Inport
  UDP Data : Inport  Port=2
  Demux : Demux  Outputs=3
  Terminator : Terminator
  Terminator1 : Terminator
  assemble robotino response : MATLAB Function  TreatAsAtomicUnit=on
  data converter : Subsystem
  v_X_lokal : Outport
  "v_Y_lokal " : Outport  Port=2
  "v_Psi_lokal " : Outport  Port=3
  "RobotinoDaten " : Outport  Port=4
  LichtschrankeGreifer : Outport  Port=5
  TasterGreifer : Outport  Port=6
  RoboID : Outport  Port=7
  wires:
  assemble robotino response/1(robotino_response) -> "RobotinoDaten "/1
  [IRDistances] -> assemble robotino response/4(distance_measuring_sensors_in)
  UDP Data/1 -> data converter/1(UDP data in)
  ProcessData/1 -> data converter/2(Robotino processed data)
  data converter/3(limit_switch_grabber) -> [limit_switch_grabber]
  data converter/1(encoder_speed) -> Demux/1
  data converter/2(light_barrier_grabber) -> [light_barrier_grabber]
  [light_barrier_grabber] -> LichtschrankeGreifer/1, assemble robotino response/6(light_barrier_in)
  [limit_switch_grabber] -> TasterGreifer/1, assemble robotino response/7(slider_in)
  data converter/4(bumper) -> [Bumper]
  data converter/5(IR_distances) -> [IRDistances]
  data converter/6(UDPmsg) -> [UDP_Msg]
  data converter/8(PowerReduction) -> Terminator1/1
  [Bumper] -> assemble robotino response/5(bumper_in)
  [vTheta] -> "v_Psi_lokal "/1, assemble robotino response/3(v_theta_in)
  [vY] -> "v_Y_lokal "/1, assemble robotino response/2(v_y_in)
  [vX] -> v_X_lokal/1, assemble robotino response/1(v_x_in)
  Demux/1 -> [vX]
  Demux/2 -> [vY]
  Demux/3 -> [vTheta]
  data converter/7(RoboID) -> RoboID/1

== system Gesamt/Regelung1/Signal Builder ==
  Demux : Demux  Tag=STV Demux  Outputs=3
  FromWs : FromWorkspace  Tag=STV FromWs  VariableName=tuvar  SampleTime=0
      SigBuilderData=|
      | common.afterFinalStr = 'Extrapolate'
      | common.sampleTime = 0
      | dataSet.timeRange = [0 25]
      | dataSet.name = 'Group 1'
      | sbobj.Groups.Name = 'Group 1'
      | sbobj.Groups.Signals(1).Name = 'X Pos'
      | sbobj.Groups.Signals(1).XData = [0 5 7.5 10 12.5 25]
      | sbobj.Groups.Signals(1).YData = [5500 5500 6500 6500 5500 5500]
      | sbobj.Groups.Signals(2).Name = 'Y Pos'
      | sbobj.Groups.Signals(2).XData = [0 2.5 5 7.5 10 25]
      | sbobj.Groups.Signals(2).YData = [1000 1000 2000 2000 1000 1000]
      | sbobj.Groups.Signals(3).Name = 'Psi'
      | sbobj.Groups.Signals(3).XData = [0 2.5 5 7.5 10 20 25]
      | sbobj.Groups.Signals(3).YData = [0 0 3.14159265359 3.14159265359 0 0 0]
      | sbobj.Groups.TimeRange = [0 25]
  X Pos : Outport  Tag=STV Outport
  Y Pos : Outport  Tag=STV Outport  Port=2
  Psi : Outport  Tag=STV Outport  Port=3
  wires:
  Demux/3 -> Psi/1
  Demux/2 -> Y Pos/1
  Demux/1 -> X Pos/1
  FromWs/1 -> Demux/1

== system Gesamt/Regelung1/Signal Builder1 ==
  Demux : Demux  Tag=STV Demux  Outputs=3
  FromWs : FromWorkspace  Tag=STV FromWs  VariableName=tuvar  SampleTime=0
  X Pos : Outport  Tag=STV Outport
  Y Pos : Outport  Tag=STV Outport  Port=2
  Psi : Outport  Tag=STV Outport  Port=3
  wires:
  Demux/3 -> Psi/1
  Demux/2 -> Y Pos/1
  Demux/1 -> X Pos/1
  FromWs/1 -> Demux/1

== system Gesamt/Regelung1/Signal Builder2 ==
  Demux : Demux  Tag=STV Demux  Outputs=3
  FromWs : FromWorkspace  Tag=STV FromWs  VariableName=tuvar  SampleTime=0
      SigBuilderData=|
      | common.afterFinalStr = 'Extrapolate'
      | common.sampleTime = 0
      | dataSet.timeRange = [0 25]
      | dataSet.name = 'Group 1'
      | sbobj.Groups.Name = 'Group 1'
      | sbobj.Groups.Signals(1).Name = 'X Pos'
      | sbobj.Groups.Signals(1).XData = [0 2.5 5 10 12.5 25]
      | sbobj.Groups.Signals(1).YData = [5500 5500 5500 5500 5500 5500]
      | sbobj.Groups.Signals(2).Name = 'Y Pos'
      | sbobj.Groups.Signals(2).XData = [0 2.5 5 10 12.5 15 25]
      | sbobj.Groups.Signals(2).YData = [1000 1000 2000 2000 1000 1000 1000]
      | sbobj.Groups.Signals(3).Name = 'Psi'
      | sbobj.Groups.Signals(3).XData = [0 6 10 20 23.72 25]
      | sbobj.Groups.Signals(3).YData = [0 0 0 0 0 0]
      | sbobj.Groups.TimeRange = [0 25]
  X Pos : Outport  Tag=STV Outport
  Y Pos : Outport  Tag=STV Outport  Port=2
  Psi : Outport  Tag=STV Outport  Port=3
  wires:
  Demux/3 -> Psi/1
  Demux/2 -> Y Pos/1
  Demux/1 -> X Pos/1
  FromWs/1 -> Demux/1

== system Gesamt/Regelung1/Signal Builder3 ==
  Demux : Demux  Tag=STV Demux  Outputs=3
  FromWs : FromWorkspace  Tag=STV FromWs  VariableName=tuvar  SampleTime=0
      SigBuilderData=|
      | common.afterFinalStr = 'Extrapolate'
      | common.sampleTime = 0
      | dataSet.timeRange = [0 45]
      | dataSet.name = 'Group 1'
      | sbobj.Groups.Name = 'Group 1'
      | sbobj.Groups.Signals(1).Name = 'X Pos'
      | sbobj.Groups.Signals(1).XData = [0 5 10 15 20 24.95 30.05 35 40 45]
      | sbobj.Groups.Signals(1).YData = [1400 1400 1900 2400 2400 2400 2400 1900 1400 1400]
      | sbobj.Groups.Signals(2).Name = 'Y Pos'
      | sbobj.Groups.Signals(2).XData = [0 0.55 5 10 15 19.95 25 29.95 35 40 45]
      | sbobj.Groups.Signals(2).YData = [1000 1000 1500 1500 1500 1500 1250 1000 1000 1000 1000]
      | sbobj.Groups.Signals(3).Name = 'Psi'
      | sbobj.Groups.Signals(3).XData = [0 5 10 15 20 25 30 35.1 40 45]
      | sbobj.Groups.Signals(3).YData = [1.5708 1.5708 6.28318530718 3.14 0 0 -3.14159265359 3.14159265359 0 0]
      | sbobj.Groups.TimeRange = [0 45]
  X Pos : Outport  Tag=STV Outport
  Y Pos : Outport  Tag=STV Outport  Port=2
  Psi : Outport  Tag=STV Outport  Port=3
  wires:
  FromWs/1 -> Demux/1
  Demux/1 -> X Pos/1
  Demux/2 -> Y Pos/1
  Demux/3 -> Psi/1

== system Gesamt/Regelung1/Signal Builder4 ==
  Demux : Demux  Tag=STV Demux  Outputs=3
  FromWs : FromWorkspace  Tag=STV FromWs  VariableName=tuvar  SampleTime=0
      SigBuilderData=|
      | common.afterFinalStr = 'Extrapolate'
      | common.sampleTime = 0
      | dataSet.timeRange = [0 45]
      | dataSet.name = 'Group 1'
      | sbobj.Groups.Name = 'Group 1'
      | sbobj.Groups.Signals(1).Name = 'X Pos'
      | sbobj.Groups.Signals(1).XData = [0 5 10 15 20 24.95 30.05 35 40 45]
      | sbobj.Groups.Signals(1).YData = [3400 3400 3900 4400 4400 4400 4400 3900 3400 3400]
      | sbobj.Groups.Signals(2).Name = 'Y Pos'
      | sbobj.Groups.Signals(2).XData = [0 0.55 5 10 15 19.95 25 29.95 35 40 45]
      | sbobj.Groups.Signals(2).YData = [1000 1000 1500 1500 1500 1500 1250 1000 1000 1000 1000]
      | sbobj.Groups.Signals(3).Name = 'Psi'
      | sbobj.Groups.Signals(3).XData = [0 5 10 15 20 25 30 35.1 40 45]
      | sbobj.Groups.Signals(3).YData = [1.5708 1.5708 6.28318530718 3.14 0 0 -3.14159265359 3.14159265359 0 0]
      | sbobj.Groups.TimeRange = [0 45]
  X Pos : Outport  Tag=STV Outport
  Y Pos : Outport  Tag=STV Outport  Port=2
  Psi : Outport  Tag=STV Outport  Port=3
  wires:
  FromWs/1 -> Demux/1
  Demux/1 -> X Pos/1
  Demux/2 -> Y Pos/1
  Demux/3 -> Psi/1

== system Gesamt/Regelung1/Signal Builder5 ==
  Demux : Demux  Tag=STV Demux  Outputs=3
  FromWs : FromWorkspace  Tag=STV FromWs  VariableName=tuvar  SampleTime=0
      SigBuilderData=|
      | common.afterFinalStr = 'Extrapolate'
      | common.sampleTime = 0
      | dataSet.timeRange = [0 45]
      | dataSet.name = 'Group 1'
      | sbobj.Groups.Name = 'Group 1'
      | sbobj.Groups.Signals(1).Name = 'X Pos'
      | sbobj.Groups.Signals(1).XData = [0 5 10 15 20 24.95 30.05 35 40 45]
      | sbobj.Groups.Signals(1).YData = [5300 4850 4100 3200 2850 2250 1900 1650 1400 750]
      | sbobj.Groups.Signals(2).Name = 'Y Pos'
      | sbobj.Groups.Signals(2).XData = [0 0.55 5 10 15 19.95 25 29.95 35 40 45]
      | sbobj.Groups.Signals(2).YData = [3450 3450 3450 3450 3450 3450 3450 3450 3450 3450 3450]
      | sbobj.Groups.Signals(3).Name = 'Psi'
      | sbobj.Groups.Signals(3).XData = [0 5 10 15 20 25 30 35.1 40 45]
      | sbobj.Groups.Signals(3).YData = [1.57079632679 1.56 1.54 0 0 -1.57079632679 -1.5 -1.46 0 0]
      | sbobj.Groups.TimeRange = [0 45]
  X Pos : Outport  Tag=STV Outport
  Y Pos : Outport  Tag=STV Outport  Port=2
  Psi : Outport  Tag=STV Outport  Port=3
  wires:
  FromWs/1 -> Demux/1
  Demux/1 -> X Pos/1
  Demux/2 -> Y Pos/1
  Demux/3 -> Psi/1

== system Gesamt/Regelung1/Stellgrößen- beschränkung  ==
  note: in mm/sec
  note: in mm/sec
  note: in rad/sec
  vX : Inport
  vY : Inport  Port=2
  vPsi : Inport  Port=3
  enableGewerk3 : Inport  Port=4
  "Beschraenkung " : MATLAB Function  TreatAsAtomicUnit=on
  MaxStellR : Constant  Value=5
  MaxStellT : Constant  Value=400
  vXlim : Outport
  vYlim : Outport  Port=2
  vPsiLim : Outport  Port=3
  wires:
  vPsi/1 -> "Beschraenkung "/5(theta)
  vY/1 -> "Beschraenkung "/4(y)
  vX/1 -> "Beschraenkung "/3(x)
  MaxStellR/1 -> "Beschraenkung "/2(MaxStellR)
  "Beschraenkung "/3(Theta) -> vPsiLim/1
  "Beschraenkung "/2(Y) -> vYlim/1
  "Beschraenkung "/1(X) -> vXlim/1
  MaxStellT/1 -> "Beschraenkung "/1(MaxStellT)
  enableGewerk3/1 -> "Beschraenkung "/6(enableGewerk3)

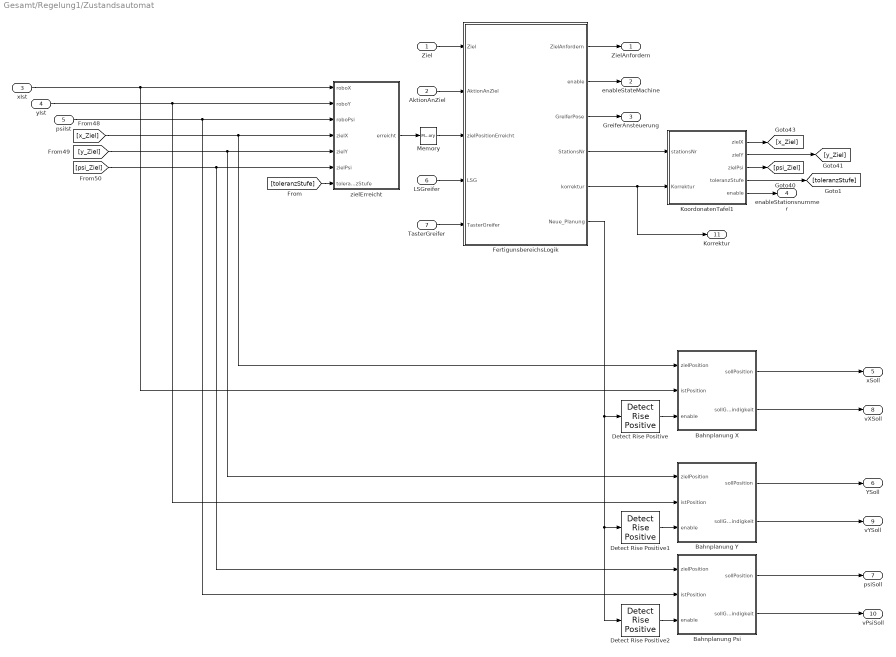
== system Gesamt/Regelung1/Zustandsautomat ==
  "Ziel " : Inport
  AktionAnZiel : Inport  Port=2
  xIst : Inport  Port=3
  yIst : Inport  Port=4
  psiIst : Inport  Port=5
  "LSGreifer " : Inport  Port=6
  "TasterGreifer " : Inport  Port=7
  Bahnplanung Psi : MATLAB Function  TreatAsAtomicUnit=on
  Bahnplanung X : MATLAB Function  TreatAsAtomicUnit=on
  Bahnplanung Y : MATLAB Function  TreatAsAtomicUnit=on
  Detect Rise Positive : simulink/Logic and Bit Operations/Detect Rise Positive  vinit=0  InputProcessing=Inherited  OutDataTypeStr=boolean
  Detect Rise Positive1 : simulink/Logic and Bit Operations/Detect Rise Positive  vinit=0  InputProcessing=Inherited  OutDataTypeStr=boolean
  Detect Rise Positive2 : simulink/Logic and Bit Operations/Detect Rise Positive  vinit=0  InputProcessing=Inherited  OutDataTypeStr=boolean
  FertigunsbereichsLogik : Stateflow chart  TreatAsAtomicUnit=on
  KoordonatenTafel1 : MATLAB Function  TreatAsAtomicUnit=on
  Memory : Memory
  zielErreicht : MATLAB Function  TreatAsAtomicUnit=on
  ZielAnfordern : Outport
  enableStateMachine : Outport  Port=2
  GreiferAnsteuerung : Outport  Port=3
  enableStationsnummer : Outport  Port=4
  xSoll : Outport  Port=5
  YSoll : Outport  Port=6
  psiSoll : Outport  Port=7
  vXSoll : Outport  Port=8
  vYSoll : Outport  Port=9
  vPsiSoll : Outport  Port=10
  Korrektur : Outport  Port=11
  wires:
  FertigunsbereichsLogik/5(korrektur) -> KoordonatenTafel1/2(Korrektur), Korrektur/1
  Bahnplanung X/2(sollGeschwindigkeit) -> vXSoll/1
  [toleranzStufe] -> zielErreicht/7(toleranzStufe)
  KoordonatenTafel1/4(toleranzStufe) -> [toleranzStufe]
  "LSGreifer "/1 -> FertigunsbereichsLogik/4(LSG)
  KoordonatenTafel1/5(enable) -> enableStationsnummer/1
  AktionAnZiel/1 -> FertigunsbereichsLogik/2(AktionAnZiel)
  FertigunsbereichsLogik/2(enable) -> enableStateMachine/1
  FertigunsbereichsLogik/4(StationsNr) -> KoordonatenTafel1/1(stationsNr)
  Memory/1 -> FertigunsbereichsLogik/3(zielPositionErreicht)
  "Ziel "/1 -> FertigunsbereichsLogik/1(Ziel)
  zielErreicht/1(erreicht) -> Memory/1
  FertigunsbereichsLogik/1(ZielAnfordern) -> ZielAnfordern/1
  FertigunsbereichsLogik/3(GreiferPose) -> GreiferAnsteuerung/1
  KoordonatenTafel1/1(zielX) -> [x_Ziel]
  KoordonatenTafel1/2(zielY) -> [y_Ziel]
  KoordonatenTafel1/3(zielPsi) -> [psi_Ziel]
  psiIst/1 -> zielErreicht/3(roboPsi), Bahnplanung Psi/2(istPosition)
  [psi_Ziel] -> zielErreicht/6(zielPsi), Bahnplanung Psi/1(zielPosition)
  yIst/1 -> zielErreicht/2(roboY), Bahnplanung Y/2(istPosition)
  [x_Ziel] -> zielErreicht/4(zielX), Bahnplanung X/1(zielPosition)
  xIst/1 -> zielErreicht/1(roboX), Bahnplanung X/2(istPosition)
  FertigunsbereichsLogik/6(Neue_Planung) -> Detect Rise Positive2/1, Detect Rise Positive1/1, Detect Rise Positive/1
  Detect Rise Positive2/1 -> Bahnplanung Psi/3(enable)
  Detect Rise Positive1/1 -> Bahnplanung Y/3(enable)
  [y_Ziel] -> zielErreicht/5(zielY), Bahnplanung Y/1(zielPosition)
  Detect Rise Positive/1 -> Bahnplanung X/3(enable)
  Bahnplanung X/1(sollPosition) -> xSoll/1
  Bahnplanung Y/1(sollPosition) -> YSoll/1
  Bahnplanung Y/2(sollGeschwindigkeit) -> vYSoll/1
  Bahnplanung Psi/1(sollPosition) -> psiSoll/1
  Bahnplanung Psi/2(sollGeschwindigkeit) -> vPsiSoll/1
  "TasterGreifer "/1 -> FertigunsbereichsLogik/5(TasterGreifer)

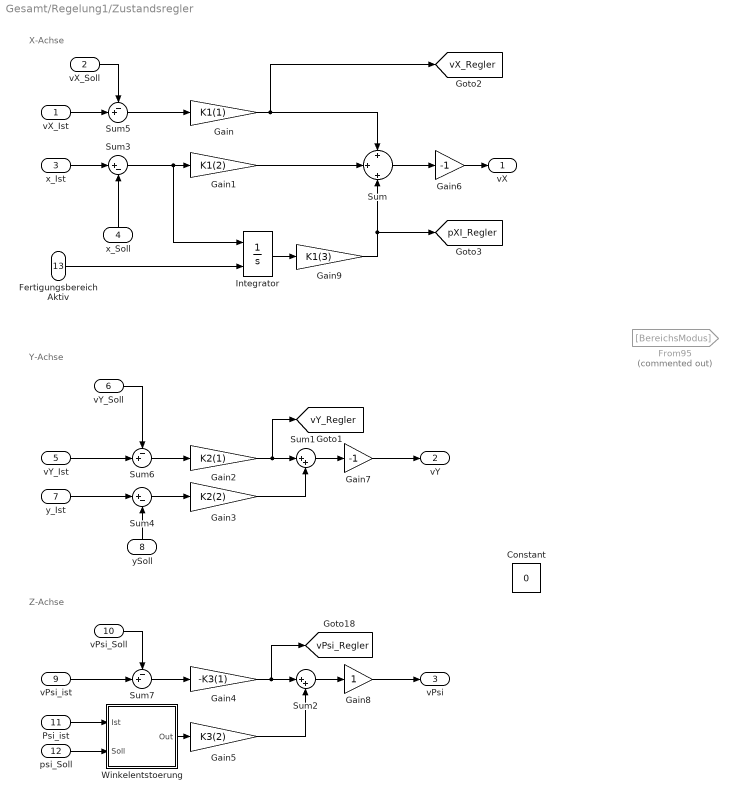
== system Gesamt/Regelung1/Zustandsregler ==
  note: X-Achse
  note: Y-Achse
  note: Z-Achse
  vX_Ist : Inport
  "vX_Soll " : Inport  Port=2
  x_Ist : Inport  Port=3
  x_Soll : Inport  Port=4
  vY_Ist : Inport  Port=5
  "vY_Soll " : Inport  Port=6
  y_Ist : Inport  Port=7
  ySoll : Inport  Port=8
  vPsi_ist : Inport  Port=9
  vPsi_Soll : Inport  Port=10
  Psi_ist : Inport  Port=11
  "psi_Soll " : Inport  Port=12
  Fertigungsbereich Aktiv : Inport  Port=13
  Constant : Constant  Value=0
  From95 : From  Commented=on  GotoTag=BereichsModus
  Gain : Gain  Gain=K1(1)
  Gain1 : Gain  Gain=K1(2)
  Gain2 : Gain  Gain=K2(1)
  Gain3 : Gain  Gain=K2(2)
  Gain4 : Gain  Gain=-K3(1)
  Gain5 : Gain  Gain=K3(2)
  Gain6 : Gain  Gain=-1
  Gain7 : Gain  Gain=-1
  Gain8 : Gain
  Gain9 : Gain  Gain=K1(3)
  Integrator : Integrator  ExternalReset=rising
  Sum : Sum  Inputs=+|+|+
  Sum1 : Sum  Inputs=|++
  Sum2 : Sum  Inputs=|++
  Sum3 : Sum  Inputs=|+-
  Sum4 : Sum  Inputs=|+-
  Sum5 : Sum  Inputs=-+|
  Sum6 : Sum  Inputs=-+|
  Sum7 : Sum  Inputs=-+|
  Winkelentstoerung : MATLAB Function  TreatAsAtomicUnit=on
  vX : Outport
  vY : Outport  Port=2
  "vPsi " : Outport  Port=3
  tag scope: pXI_Regler=global, vPsi_Regler=global, vX_Regler=global, vY_Regler=global
  wires:
  Gain9/1 -> Sum/3, [pXI_Regler]
  Integrator/1 -> Gain9/1
  Winkelentstoerung/1(Out) -> Gain5/1
  "psi_Soll "/1 -> Winkelentstoerung/2(Soll)
  ySoll/1 -> Sum4/2
  x_Soll/1 -> Sum3/2
  vPsi_Soll/1 -> Sum7/1
  Sum7/1 -> Gain4/1
  "vY_Soll "/1 -> Sum6/1
  "vX_Soll "/1 -> Sum5/1
  Sum6/1 -> Gain2/1
  vY_Ist/1 -> Sum6/2
  Sum5/1 -> Gain/1
  vX_Ist/1 -> Sum5/2
  Psi_ist/1 -> Winkelentstoerung/1(Ist)
  Gain8/1 -> "vPsi "/1
  Sum2/1 -> Gain8/1
  vPsi_ist/1 -> Sum7/2
  Gain7/1 -> vY/1
  Gain6/1 -> vX/1
  Sum4/1 -> Gain3/1
  y_Ist/1 -> Sum4/1
  Sum3/1 -> Gain1/1, Integrator/1
  x_Ist/1 -> Sum3/1
  Sum/1 -> Gain6/1
  Sum1/1 -> Gain7/1
  Gain5/1 -> Sum2/2
  Gain4/1 -> [vPsi_Regler], Sum2/1
  Gain3/1 -> Sum1/2
  Gain2/1 -> Sum1/1, [vY_Regler]
  Gain1/1 -> Sum/2
  Gain/1 -> Sum/1, [vX_Regler]
  Fertigungsbereich Aktiv/1 -> Integrator/2

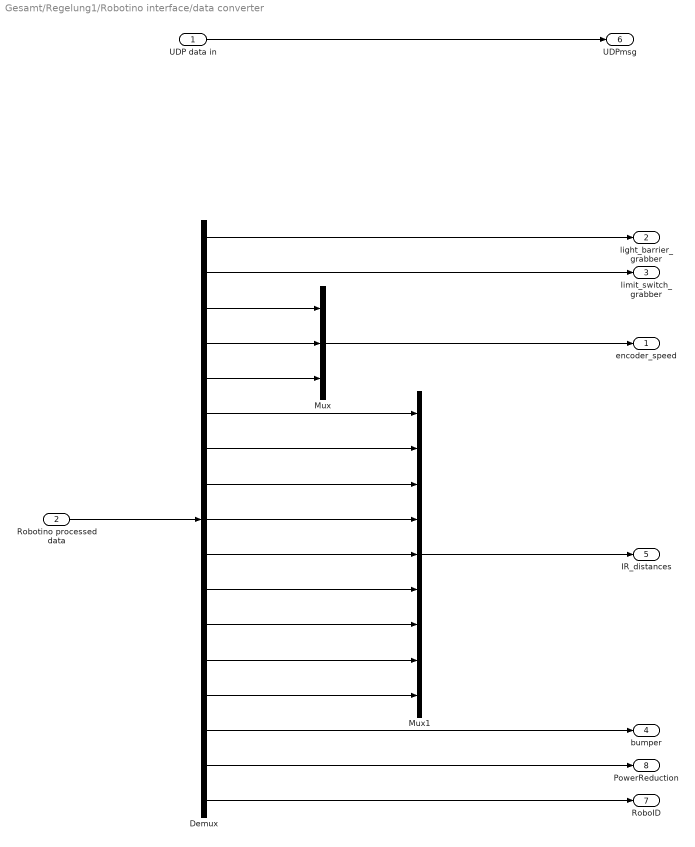
== system Gesamt/Regelung1/Robotino interface/data converter ==
  UDP data in : Inport
  Robotino processed data : Inport  Port=2
  Demux : Demux  Outputs=17
  Mux : Mux  Inputs=3
  Mux1 : Mux  Inputs=9
  encoder_speed : Outport
  light_barrier_grabber : Outport  Port=2
  limit_switch_grabber : Outport  Port=3
  bumper : Outport  Port=4
  IR_distances : Outport  Port=5
  UDPmsg : Outport  Port=6
  RoboID : Outport  Port=7
  PowerReduction : Outport  Port=8
  wires:
  Demux/15 -> bumper/1
  Mux1/1 -> IR_distances/1
  Demux/14 -> Mux1/9
  Demux/13 -> Mux1/8
  Demux/12 -> Mux1/7
  Demux/11 -> Mux1/6
  Demux/10 -> Mux1/5
  Demux/9 -> Mux1/4
  Demux/8 -> Mux1/3
  Demux/6 -> Mux1/1
  Demux/7 -> Mux1/2
  Mux/1 -> encoder_speed/1
  Demux/5 -> Mux/3
  Demux/4 -> Mux/2
  Demux/3 -> Mux/1
  Demux/2 -> limit_switch_grabber/1
  Demux/1 -> light_barrier_grabber/1
  Robotino processed data/1 -> Demux/1
  UDP data in/1 -> UDPmsg/1
  Demux/17 -> RoboID/1
  Demux/16 -> PowerReduction/1

== stateflow chart Gesamt/Bahnplanung1/Auftrags_Koordination ==
  settings: updateMethod=DISCRETE  sampleTime=dt
  state Auftragskoordination
    state WerkstueckAufgenommen
      entry:Werkstueck=1,
      AktuellesZiel=ZielPos,
      Bearbeitet=1;
    state KeinWerkstueckAufgenommen
      entry:Werkstueck=0,
      AktuellesZiel=WerkstueckPos,
      Bearbeitet=1;
    state AufAuftragWarten
      entry:Werkstueck=0,
      AktuellesZiel=100
      Bearbeitet=0;
    KeinWerkstueckAufgenommen -> WerkstueckAufgenommen : [Werkstueckerkannt==1 && Transportbereich==1]
    WerkstueckAufgenommen -> AufAuftragWarten : [Werkstueckerkannt==0 && Transportbereich==1]
    AufAuftragWarten -> KeinWerkstueckAufgenommen : [NeuerAuftrag]
    (default) -> AufAuftragWarten
  data: NeuerAuftrag input; WerkstueckPos input; ZielPos input; AktuellesZiel output; Werkstueck output; Werkstueckerkannt input; Transportbereich input; Bearbeitet output

== stateflow chart Gesamt/Bahnplanung1/Fifo Steuerung/Fifo ==
  settings: updateMethod=DISCRETE  sampleTime=dt
  state FIFOStationen
    state Auftrag_Roboter_1
    state Zielbereich_untersuchen
      entry:
      ersterFifo=floor(Zielstation/2)*3+2*mod(Zielstation,2)+1;
    state Fifo_einfachbesetzt1
      entry:
      zweiterFifo=floor(Zielstation/2)*3+1+1;
      Fifo=2;
    state Fifo_frei
      entry:
      Fifo=1;
    state Fifo_doppelt_besetzt
      entry:
      dritterFifo=floor(Zielstation/2)*3+2-2*mod(Zielstation,2)+1;
      Fifo=3;
    state Fifo_voll
      entry:
      Fifo=4;
    state Uebergabepunkt_gleich_Zielpunkt
      entry:
      Fifo=0;
    (default) -> Auftrag_Roboter_1
    Auftrag_Roboter_1 -> Zielbereich_untersuchen : [Zielposition>-1]
    Zielbereich_untersuchen -> Fifo_einfachbesetzt1 [order 1] : [(FifoArray(ersterFifo)~=0)| (FifoArray(ersterFifo)==0 & StationArray(Zielstation+1)~=0) ]
    Uebergabepunkt_gleich_Zielpunkt -> Zielbereich_untersuchen
    Zielbereich_untersuchen -> Uebergabepunkt_gleich_Zielpunkt [order 2]
    Fifo_einfachbesetzt1 -> Fifo_frei [order 2] : [FifoArray(ersterFifo)==0]
    Fifo_einfachbesetzt1 -> Fifo_doppelt_besetzt [order 1] : [(FifoArray(zweiterFifo)~=0)]
    Fifo_doppelt_besetzt -> Fifo_voll [order 2] : [(FifoArray(dritterFifo)~=0)]
    Fifo_frei -> Uebergabepunkt_gleich_Zielpunkt : [ StationArray(Zielstation+1)==0]
    Fifo_doppelt_besetzt -> Fifo_einfachbesetzt1 [order 1] : [FifoArray(zweiterFifo)==0]
    Fifo_voll -> Fifo_doppelt_besetzt : [FifoArray(dritterFifo)==0]
  state Wartebereich
    entry: Fifo=4;
  state Ladestation
    entry: Fifo=0;
  (default) -> Wartebereich
  Wartebereich -> FIFOStationen [order 1] : [Zielstation<8]
  FIFOStationen -> Wartebereich [order 1] : [Zielstation==10]
  Ladestation -> Wartebereich [order 1] : [Zielstation==10]
  Wartebereich -> Ladestation [order 2] : [Zielstation>=8 & Zielstation<10]
  Ladestation -> FIFOStationen [order 2] : [Zielstation<8]
  FIFOStationen -> Ladestation [order 2] : [Zielstation>=8 & Zielstation<10]
  data: FifoArray input; Zielposition input; Zielstation input; Fifo output; StationArray input; dritterFifo local; zweiterFifo local; ersterFifo local

== matlab function Gesamt/Bahnplanung1/Fifo Steuerung/Positionszuweisung ==
  data: Fifo input; Zielstation input; Endposition output; RoboterID input
function Endposition = fcn(Fifo,Zielstation,RoboterID)
Endposition=zeros([1 2]);

WartepositionX= 6311;
WartepositionY=[550 950 1350 1750 2150];

StationvorneX=[853 1361 2058 2559 3256 3762 4448 4953 6311 6311];
StationvorneY=[2300 2300 2300 2300 2300 2300 2300 2300 2592 3080];
%Stationhinten=[856 1364 2059 2560 3259 3763 4451 4958];

ersterFifo=floor(Zielstation/2)*3+2*mod(Zielstation,2);
zweiterFifo=floor(Zielstation/2)*3+1;
dritterFifo=floor(Zielstation/2)*3+2-2*mod(Zielstation,2);

if Fifo==0
    Endposition(1)=StationvorneX(Zielstation+1);
    Endposition(2)=StationvorneY(Zielstation+1);
    else if Fifo==1
        Endposition(1)= ersterFifo*400+703;
        Endposition(2)= 250;
       
    else if Fifo==2
            Endposition(1)= zweiterFifo*400+703;
            Endposition(2)= 250;
        
    else if Fifo==3
            Endposition(1)= dritterFifo*400+703;
            Endposition(2)= 250;
            else
            Endposition(2)= WartepositionY(RoboterID);
            Endposition(1)= WartepositionX;
        end
        end
        end
end
end

== matlab function Gesamt/Bahnplanung1/Fifo Steuerung/ZielPosSplitten ==
  data: AktuellesZiel input; ZielPos output; Zielstation output
function [ZielPos,Zielstation]= fcn(AktuellesZiel)
ZielPos=mod(AktuellesZiel,10);
Zielstation=round(AktuellesZiel/10);

== matlab function Gesamt/Bahnplanung1/Fifo Steuerung/ZielStation_Erreicht ==
  data: Erreicht output; AktuellePos input; Zielpos input
function Erreicht = fcn(AktuellePos,Zielpos)
Abstand=sqrt((AktuellePos(1)-Zielpos(1))^2+(AktuellePos(2)-Zielpos(2))^2);
%S=round((X-900)/560);
if AktuellePos(2) >2000 && AktuellePos(2)<2500&& AktuellePos(1)>600 && AktuellePos(1) < 5200 && Abstand < 150
    Erreicht=1;
else
    Erreicht=0;
end
end
